simulink model "rrtm"  (R2024b)
settings: Solver=VariableStepAuto  StartTime=0.0  StopTime=inf  RelTol=1e-3
values from neighbouring files (symbols this model uses):
  waypoint = zeros(size(pathObj.States, 1),2)    [astar.m]    (also in rrt-son.m; rrt.m; rrtson.m)
undefined symbols (not defined in the file or in its folder): Angular, Linear
libraries: robotlib x3, robotalgslib x1
settings Model: Creator=a_met  LastModifiedBy=a_met

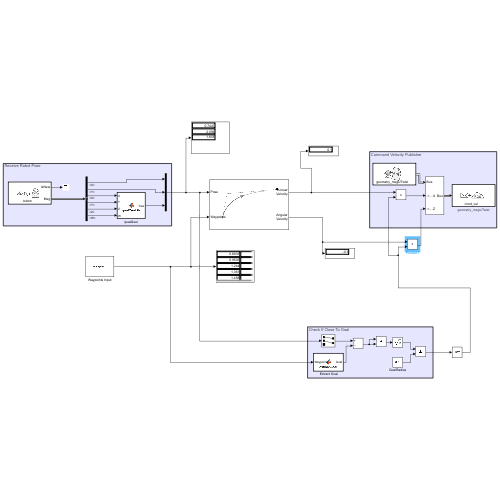
[thumbnail: Simulink's stored preview of the top-level diagram]
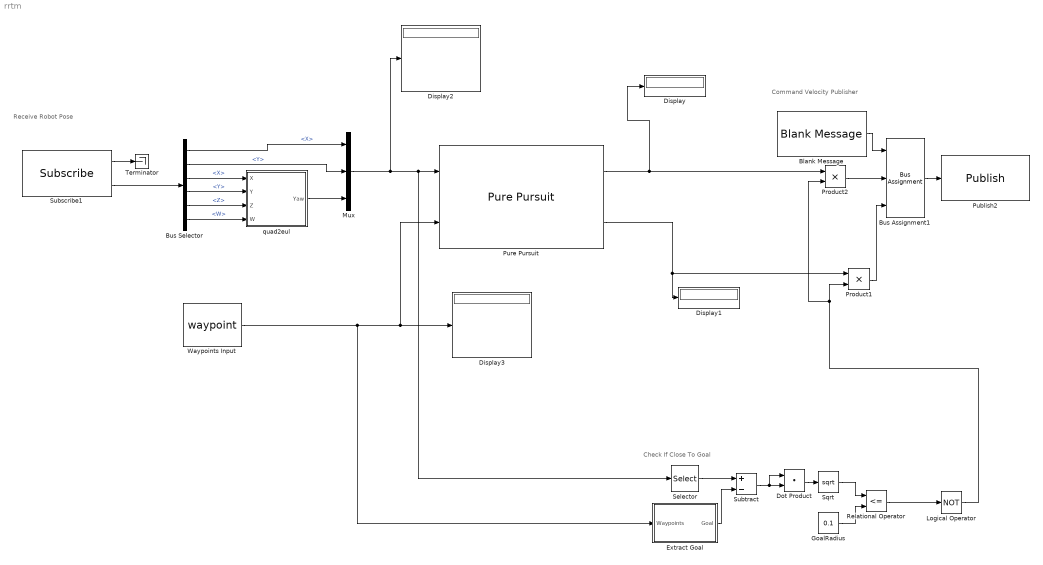
== system rrtm ==
  note: Receive Robot Pose
  note: Command Velocity Publisher
  note: Check If Close To Goal
  " Extract Goal" : MATLAB Function  TreatAsAtomicUnit=on
  Blank Message : robotlib/Blank Message  messageClass=Message  entityType=geometry_msgs/Twist  messageType=geometry_msgs/Twist  SampleTime=inf  legacyBusStruct=off
  Bus Assignment1 : BusAssignment  DialogController=Simulink.DDGSource_BusAssignment  AssignedSignals=Linear.X,Angular.Z
  Bus Selector : BusSelector  OutputSignals=Pose.Pose.Position.X,Pose.Pose.Position.Y,Pose.Pose.Orientation.X,Pose.Pose.Orientation.Y,Pose.Pose.Orientation.Z,Pose.Pose.Orientation.W
  Display{,1..3} (4 alike) : Display
  Dot Product : DotProduct  OutDataTypeStr=Inherit: Inherit via internal rule
  GoalRadius : Constant  Value=0.1
  Logical Operator : Logic  Operator=NOT  AllPortsSameDT=off  OutDataTypeStr=boolean
  Mux : Mux  Inputs=3
  Product1 : Product
  Product2 : Product
  Publish2 : robotlib/Publish  topicSource=Select from ROS network  topic=/cmd_vel  messageType=geometry_msgs/Twist  legacyBusStruct=off  messageQueueLength=105
  Pure Pursuit : robotalgslib/Pure Pursuit  DesiredLinearVelocityPort=off  DesiredLinearVelocity=0.1  MaxAngularVelocity=0.3  LookaheadDistancePort=off  LookaheadDistance=0.03  TargetDirPort=off  SimulateUsing=Code generation
      settings: LibrarySourceBlock=robotmobilelib/Pure Pursuit
  Relational Operator : RelationalOperator  Operator=<=  OutDataTypeStr=boolean  RndMeth=Simplest  InputSameDT=off
  Selector : Selector  InputPortWidth=3  IndexOptions=Index vector (dialog)  Indices=[1 2]  OutputSizes=1
  Sqrt : Sqrt
  Subscribe1 : robotlib/Subscribe  topicSource=Select from ROS network  topic=/odom  messageType=nav_msgs/Odometry  SampleTime=-1  legacyBusStruct=off  messageQueueLength=1
  Subtract : Sum  Inputs=+-
  Terminator : Terminator
  Waypoints Input : Constant  Value=waypoint  VectorParams1D=off  OutDataTypeStr=double
  quad2eul : MATLAB Function  TreatAsAtomicUnit=on
  wires:
  Bus Selector/1 -> Mux/1  "<X>"
  quad2eul/1(Yaw) -> Mux/3
  Bus Selector/2 -> Mux/2  "<Y>"
  Mux/1 -> Display2/1, Selector/1, Pure Pursuit/1
  Subscribe1/2 -> Bus Selector/1
  Bus Selector/3 -> quad2eul/1(X)  "<X>"
  Bus Selector/4 -> quad2eul/2(Y)  "<Y>"
  Subscribe1/1 -> Terminator/1
  Bus Selector/5 -> quad2eul/3(Z)  "<Z>"
  Blank Message/1 -> Bus Assignment1/1
  Pure Pursuit/1 -> Product2/1, Display/1
  Bus Assignment1/1 -> Publish2/1
  Pure Pursuit/2 -> Product1/1, Display1/1
  Waypoints Input/1 -> " Extract Goal"/1(Waypoints), Pure Pursuit/2, Display3/1
  Bus Selector/6 -> quad2eul/4(W)  "<W>"
  Relational Operator/1 -> Logical Operator/1
  " Extract Goal"/1(Goal) -> Subtract/2
  Dot Product/1 -> Sqrt/1
  Sqrt/1 -> Relational Operator/1
  Selector/1 -> Subtract/1
  Subtract/1 -> Dot Product/1, Dot Product/2
  GoalRadius/1 -> Relational Operator/2
  Logical Operator/1 -> Product2/2, Product1/2
  Product1/1 -> Bus Assignment1/3
  Product2/1 -> Bus Assignment1/2

== matlab function rrtm/quad2eul ==
  data: X input; Yaw output; Y input; Z input; W input
function Yaw = quat2eulBlk(X, Y, Z, W)
%#codegen

eularAngles = quat2eul([W, X, Y, Z]);
Yaw = eularAngles(1);

== matlab function rrtm/ Extract Goal ==
  data: Waypoints input; Goal output
function Goal = extractGoal(Waypoints)
%#codegen
b = isnan(Waypoints);
[rows,~] = find(b);
ridx = setdiff(1:size(Waypoints,1), sort(rows));
Goal = [Waypoints(ridx(end), 1) Waypoints(ridx(end), 2)];
